simulink model "tests"  (Simulink 8.1)
settings: Solver=FixedStepDiscrete  StartTime=0.0  StopTime=10  FixedStep=0.05  RelTol=1e-3
libraries: simulink x1, rtwinlib x1
Description:
  | Vectorized Quantizer C-MEX S-function
settings Model: Creator=The MathWorks Inc.  LastModifiedBy=ARAS_Robotic1  ExtModeTrigMode=oneshot  ExtModeArmWhenConnect=off
settings SolverCC: PositivePriorityOrder=on
settings DataIOCC: LimitDataPoints=off
settings OptimizationCC: BlockReduction=off  BooleanDataType=off  InitFltsAndDblsToZero=on
settings DebuggingCC: SaveWithParameterizedLinksMsg=none  SignalResolutionControl=TryResolveAllWithWarning  SolverPrmCheckMsg=none  MultiTaskDSMMsg=warning  MultiTaskCondExecSysMsg=none
settings HardwareCC: ProdIntDivRoundTo=Zero  ProdEndianess=LittleEndian  ProdHWDeviceType=Generic->32-bit x86 compatible  TargetIntDivRoundTo=Zero  TargetEndianess=LittleEndian  TargetHWDeviceType=MATLAB Host  ProdEqTarget=off
settings SFSimCC: SimCustomHeaderCode=|
  | advapi32.dll
  | comctl32.dll
  | comdlg32.dll
  | gdi32.dll
  | kernel32.dll
  | netapi32.dll
  | shell32.dll
  | shlwapi.dll
  | user32.dll
  | WindowsCodecs.dll
settings SFSimCC: SimUserLibraries=|
  | NtDsAPI.Lib
  | NTMSAPI.Lib
  | NtQuery.Lib
  | windowscodecs.lib
settings RTWCC: ProcessScript=grt_make_rtw_hook  CustomLibrary=kernel32.lib  IncludeERTFirstTime=on  RTWCompilerOptimization=On
settings CodeAppCC: MaxIdLength=95
settings GRTTargetCC: CombineOutputUpdateFcns=on  GRTInterface=off

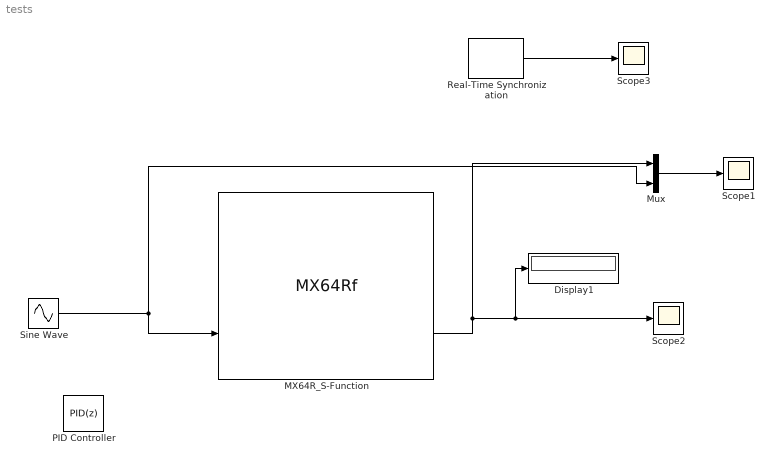
== system tests ==
  Display1 : Display
  MX64R_S-Function : S-Function  FunctionName=MX64Rf  Parameters=p1,p2,p3,p4  EnableBusSupport=off  mask(S-function: MX64R){p1=1, p2=2000000, p3=3, p4=6}
      mask prompts: p1 "Port Num"; p2 "Boad Rate"; p3 "Dynamixel ID"; p4 "methode"
      mask help:
      | this Block is desined for position and torque control of MX64R Dynamixel
      | copyright @ Aras Lab.
      mask Display:
      | image('mx64RR.jpg')
      | port_label('input',1,'desire_torque')
      | port_label('input',2,'desire_position')
      | port_label('output',1,'current_load')
      | port_label('output',2,'current_position')
  Mux : Mux  Inputs=2
  PID Controller : simulink/Continuous/PID Controller  Controller=PID  TimeDomain=Discrete-time  SampleTime=-1  IntegratorMethod=Forward Euler  FilterMethod=Forward Euler  Form=Parallel  P=1  I=1  D=0  N=100  InitialConditionSource=internal  InitialConditionForIntegrator=0  InitialConditionForFilter=0  ExternalReset=none  LimitOutput=off  UpperSaturationLimit=inf  LowerSaturationLimit=-inf  LinearizeAsGain=on  AntiWindupMode=none  Kb=1  TrackingMode=off  Kt=1  PParamMin=[]  PParamMax=[]  IParamMin=[]  IParamMax=[]  DParamMin=[]  DParamMax=[]  NParamMin=[]  NParamMax=[]  KbParamMin=[]  KbParamMax=[]  KtParamMin=[]  KtParamMax=[]  POutMin=[]  POutMax=[]  IOutMin=[]  IOutMax=[]  DOutMin=[]  DOutMax=[]  NOutMin=[]  NOutMax=[]  KbOutMin=[]  KbOutMax=[]  KtOutMin=[]  KtOutMax=[]  IntegratorOutMin=[]  IntegratorOutMax=[]  FilterOutMin=[]  FilterOutMax=[]  SumOutMin=[]  SumOutMax=[]  SumI1OutMin=[]  SumI1OutMax=[]  SumI2OutMin=[]  SumI2OutMax=[]  SumI3OutMin=[]  SumI3OutMax=[]  SumDOutMin=[]  SumDOutMax=[]  SaturationOutMin=[]  SaturationOutMax=[]  IntegratorContinuousStateAttributes=''  IntegratorStateMustResolveToSignalObject=off  IntegratorRTWStateStorageClass=Auto  FilterContinuousStateAttributes=''  FilterStateMustResolveToSignalObject=off  FilterRTWStateStorageClass=Auto
  Real-Time Synchronization : rtwinlib/Real-Time Synchronization  SampleTime=0.05  MaxMissedTicks=10000  ShowMissedTicks=on  YieldWhenWaiting=off
  Scope1 : Scope
      settings: YMin=-0.5  YMax=6.5  SaveName=ScopeData2
  Scope2 : Scope
      settings: YMin=-0.5  YMax=6.5
  Scope3 : Scope
      settings: TimeRange=10  YMin=35  YMax=135
  Sine Wave : Sin  Bias=1
  wires:
  MX64R_S-Function/2 -> Display1/1, Scope2/1, Mux/1
  Mux/1 -> Scope1/1
  Real-Time Synchronization/1 -> Scope3/1
  Sine Wave/1 -> MX64R_S-Function/2, Mux/2
